simulink model "JuntaFexible"  (R2015a)
settings: Solver=ode4  StartTime=0.0  StopTime=10.0  FixedStep=.001  RelTol=1e-3
settings Model: Creator=Alberto  LastModifiedBy=Jesus
settings DataIOCC: SignalLoggingSaveFormat=ModelDataLogs
settings DebuggingCC: UnderspecifiedInitializationDetection=Classic  MergeDetectMultiDrivingBlocksExec=none  SolverPrmCheckMsg=warning  MultiTaskDSMMsg=warning  MultiTaskCondExecSysMsg=none  StateNameClashWarn=warning

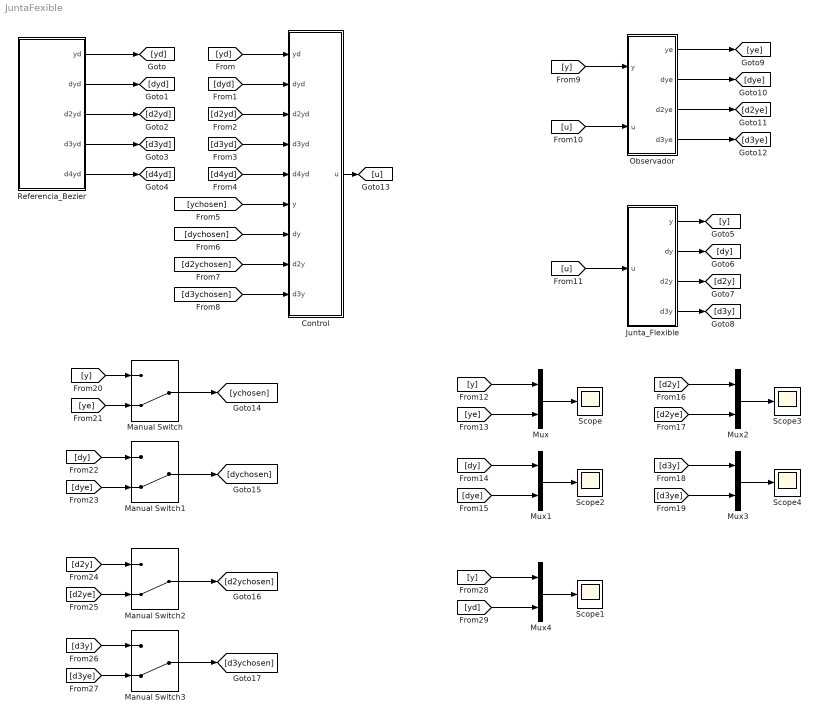
== system JuntaFexible ==
  Control : Subsystem  mask{K=.8, Jl=.1, Jm=.1, Bl=.001, Bm=0.015, z1=5, z2=7.5, w1=150, w2=175}
      mask init:
      | a4=Jl*Jm;
      | a3=Jl*Bm+Jm*Bl;
      | a2=K*(Jl+Jm)+Bl*Bm;
      | a1=K*(Bl+Bm);
      | PD=conv([1 2*z1*w1 w1^2],[1 2*z2*w2 w2^2]);
      | k3=PD(2)-(a3/a4);
      | k2=PD(3)-(a2/a4);
      | k1=PD(4)-(a1/a4);
      | k0=PD(5);
  Junta_Flexible : Subsystem  mask{K=0.8, Jl=.1, Jm=.1, Bl=.001, Bm=.015, y0=.4, dy0=.5, d2y0=0, d3y0=0}
  Manual Switch{,1..3} (4 alike) : ManualSwitch  CurrentSetting=0
  Mux{,1..4} (5 alike) : Mux  Inputs=2
  Observador : Subsystem  mask{K=0.8, Jl=.1, Jm=.1, Bl=.001, Bm=.015, z1o=1, z2o=2, w1o=10, w2o=15}
      mask prompts: z2o "z20"
      mask init:
      | alpha2=K*(Bl+Bm)/(Jl*Jm);
      | alpha3=(K/Jl)+(K/Jm)+((Bl*Bm)/(Jl*Jm));
      | alpha4=(Bl/Jl)+(Bm/Jm);
      | beta=K/(Jl*Jm);
      | PD=conv([1 2*z1o*w1o w1o^2],[1 2*z2o*w2o w2o^2]);
      | lambda3=PD(2)-alpha4;
      | lambda2=PD(3)-alpha3-alpha4*lambda3;
      | lambda1=PD(4)-alpha2-alpha3*lambda3-alpha4*lambda2;
      | lambda0=PD(5)-alpha2*lambda3-alpha3*lambda2-alpha4*lambda1;
  Referencia_Bezier : Subsystem  mask{t1=2, t2=4, y0=.1, yf=10}
      mask prompts: y0 "Valor Inicial"; yf "Valor final"
      mask init:
      | A=[1 -1 1 -1 1;...
      |     5 -6 7 -8 9;...
      |     20 -30 42 -56 72;...
      |     60 -120 210 -336 504;...
      |     120 -360 840 -1680 3024];
      | B=[1;0;0;0;0];
      | x=inv(A)*B;
      | gamma1=x(1)
      | gamma2=x(2)
      | gamma3=x(3)
      | gamma4=x(4)
      | gamma5=x(5)
  Scope{,1..4} (5 alike) : Scope
      Scope settings: YMin=-1  YMax=12
      Scope1 settings: YMin=-1.38898  YMax=11.26544
      Scope2 settings: YMin=-1  YMax=12  SaveName=ScopeData2
      Scope3 settings: YMin=-130.40405  YMax=113.50003  SaveName=ScopeData3
      Scope4 settings: YMin=-367942.44454  YMax=367940.37596  SaveName=ScopeData4
  wires:
  Mux/1 -> Scope/1
  Referencia_Bezier/1(yd) -> [yd]
  Referencia_Bezier/2(dyd) -> [dyd]
  Referencia_Bezier/3(d2yd) -> [d2yd]
  Referencia_Bezier/4(d3yd) -> [d3yd]
  Referencia_Bezier/5(d4yd) -> [d4yd]
  [yd] -> Control/1(yd)
  [dyd] -> Control/2(dyd)
  [d2yd] -> Control/3(d2yd)
  [d3yd] -> Control/4(d3yd)
  [d4yd] -> Control/5(d4yd)
  Junta_Flexible/1(y) -> [y]
  Junta_Flexible/2(dy) -> [dy]
  Junta_Flexible/3(d2y) -> [d2y]
  Junta_Flexible/4(d3y) -> [d3y]
  [ychosen] -> Control/6(y)
  [dychosen] -> Control/7(dy)
  [d2ychosen] -> Control/8(d2y)
  [d3ychosen] -> Control/9(d3y)
  [y] -> Observador/1(y)
  [u] -> Observador/2(u)
  Observador/1(ye) -> [ye]
  Observador/2(dye) -> [dye]
  Observador/3(d2ye) -> [d2ye]
  Observador/4(d3ye) -> [d3ye]
  Control/1(u) -> [u]
  [u] -> Junta_Flexible/1(u)
  [y] -> Mux/1
  [ye] -> Mux/2
  Mux1/1 -> Scope2/1
  [dy] -> Mux1/1
  [dye] -> Mux1/2
  Mux2/1 -> Scope3/1
  [d2y] -> Mux2/1
  [d2ye] -> Mux2/2
  Mux3/1 -> Scope4/1
  [d3y] -> Mux3/1
  [d3ye] -> Mux3/2
  [y] -> Manual Switch/1
  [ye] -> Manual Switch/2
  Manual Switch/1 -> [ychosen]
  Manual Switch1/1 -> [dychosen]
  [dy] -> Manual Switch1/1
  [dye] -> Manual Switch1/2
  Manual Switch2/1 -> [d2ychosen]
  Manual Switch3/1 -> [d3ychosen]
  [d2y] -> Manual Switch2/1
  [d2ye] -> Manual Switch2/2
  [d3y] -> Manual Switch3/1
  [d3ye] -> Manual Switch3/2
  Mux4/1 -> Scope1/1
  [y] -> Mux4/1
  [yd] -> Mux4/2

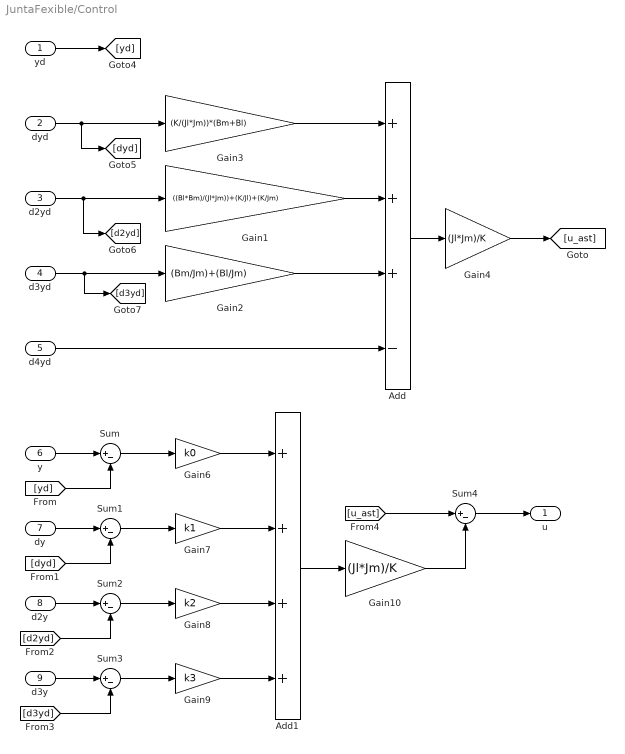
== system JuntaFexible/Control ==
  yd : Inport
  dyd : Inport  Port=2
  d2yd : Inport  Port=3
  d3yd : Inport  Port=4
  d4yd : Inport  Port=5
  y : Inport  Port=6
  dy : Inport  Port=7
  d2y : Inport  Port=8
  d3y : Inport  Port=9
  Add : Sum  Inputs=+++-
  Add1 : Sum  Inputs=++++
  Gain1 : Gain  Gain=((Bl*Bm)/(Jl*Jm))+(K/Jl)+(K/Jm)
  Gain10 : Gain  Gain=(Jl*Jm)/K
  Gain2 : Gain  Gain=(Bm/Jm)+(Bl/Jm)
  Gain3 : Gain  Gain=(K/(Jl*Jm))*(Bm+Bl)
  Gain4 : Gain  Gain=(Jl*Jm)/K
  Gain6 : Gain  Gain=k0
  Gain7 : Gain  Gain=k1
  Gain8 : Gain  Gain=k2
  Gain9 : Gain  Gain=k3
  Sum{,1..4} (5 alike) : Sum  Inputs=|+-
  u : Outport
  wires:
  d3yd/1 -> [d3yd], Gain2/1
  d2yd/1 -> [d2yd], Gain1/1
  Gain1/1 -> Add/2
  Gain2/1 -> Add/3
  Add/1 -> Gain4/1
  dyd/1 -> Gain3/1, [dyd]
  Gain3/1 -> Add/1
  Gain4/1 -> [u_ast]
  yd/1 -> [yd]
  y/1 -> Sum/1
  [yd] -> Sum/2
  Sum/1 -> Gain6/1
  dy/1 -> Sum1/1
  [dyd] -> Sum1/2
  Sum1/1 -> Gain7/1
  d2y/1 -> Sum2/1
  [d2yd] -> Sum2/2
  d3y/1 -> Sum3/1
  [d3yd] -> Sum3/2
  Sum2/1 -> Gain8/1
  Sum3/1 -> Gain9/1
  Gain6/1 -> Add1/1
  Gain7/1 -> Add1/2
  Gain8/1 -> Add1/3
  Gain9/1 -> Add1/4
  Add1/1 -> Gain10/1
  [u_ast] -> Sum4/1
  Gain10/1 -> Sum4/2
  Sum4/1 -> u/1
  d4yd/1 -> Add/4

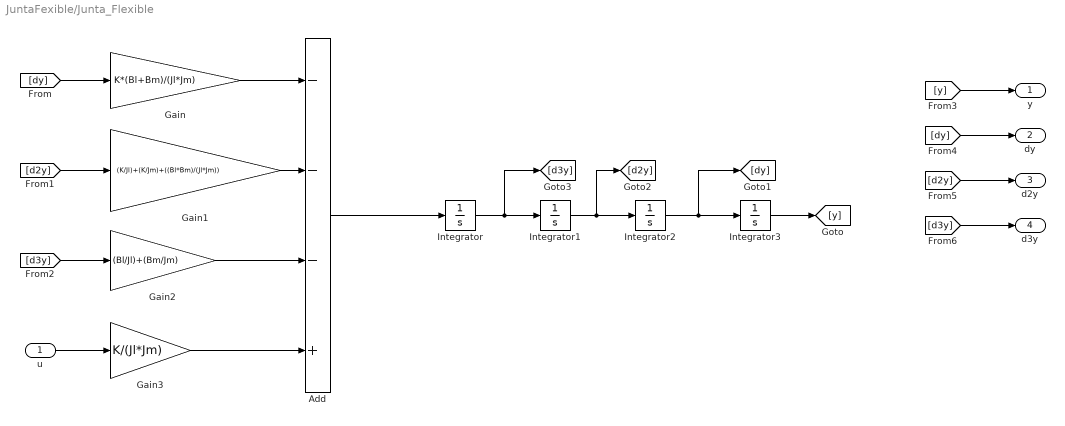
== system JuntaFexible/Junta_Flexible ==
  u : Inport
  Add : Sum  Inputs=---+
  Gain : Gain  Gain=K*(Bl+Bm)/(Jl*Jm)
  Gain1 : Gain  Gain=(K/Jl)+(K/Jm)+((Bl*Bm)/(Jl*Jm))
  Gain2 : Gain  Gain=(Bl/Jl)+(Bm/Jm)
  Gain3 : Gain  Gain=K/(Jl*Jm)
  Integrator : Integrator  InitialCondition=d3y0
  Integrator1 : Integrator  InitialCondition=d2y0
  Integrator2 : Integrator  InitialCondition=dy0
  Integrator3 : Integrator  InitialCondition=y0
  y : Outport
  dy : Outport  Port=2
  d2y : Outport  Port=3
  d3y : Outport  Port=4
  wires:
  Integrator3/1 -> [y]
  Integrator/1 -> [d3y], Integrator1/1
  [d3y] -> d3y/1
  Gain/1 -> Add/1
  [y] -> y/1
  Integrator2/1 -> [dy], Integrator3/1
  Integrator1/1 -> [d2y], Integrator2/1
  [dy] -> Gain/1
  Gain2/1 -> Add/3
  Gain3/1 -> Add/4
  Gain1/1 -> Add/2
  [dy] -> dy/1
  [d2y] -> d2y/1
  [d2y] -> Gain1/1
  Add/1 -> Integrator/1
  [d3y] -> Gain2/1
  u/1 -> Gain3/1

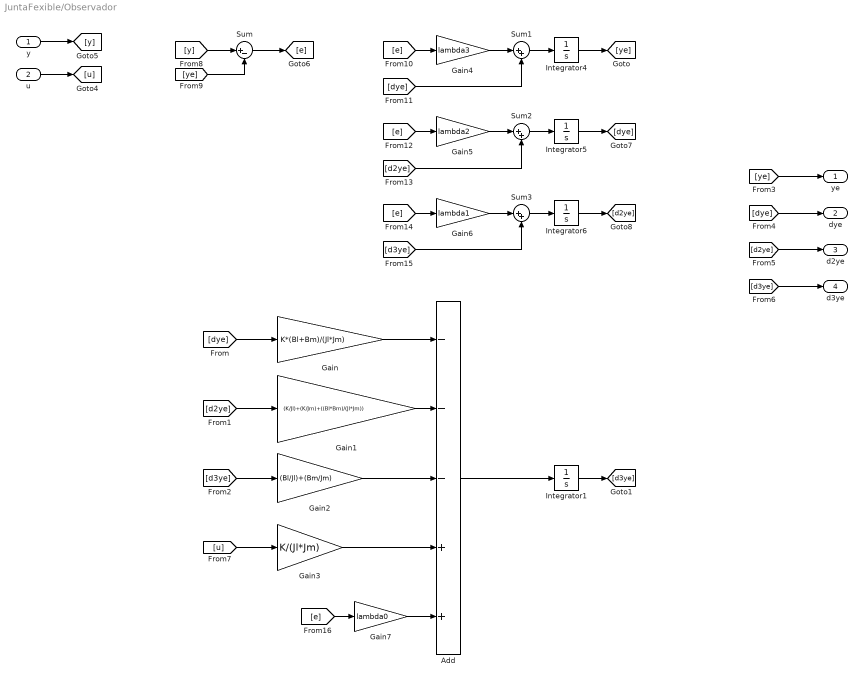
== system JuntaFexible/Observador ==
  y : Inport
  u : Inport  Port=2
  Add : Sum  Inputs=---++
  Gain : Gain  Gain=K*(Bl+Bm)/(Jl*Jm)
  Gain1 : Gain  Gain=(K/Jl)+(K/Jm)+((Bl*Bm)/(Jl*Jm))
  Gain2 : Gain  Gain=(Bl/Jl)+(Bm/Jm)
  Gain3 : Gain  Gain=K/(Jl*Jm)
  Gain4 : Gain  Gain=lambda3
  Gain5 : Gain  Gain=lambda2
  Gain6 : Gain  Gain=lambda1
  Gain7 : Gain  Gain=lambda0
  Integrator{1,4..6} (4 alike) : Integrator
  Sum : Sum  Inputs=|+-
  Sum1 : Sum  Inputs=|++
  Sum2 : Sum  Inputs=|++
  Sum3 : Sum  Inputs=|++
  ye : Outport
  dye : Outport  Port=2
  d2ye : Outport  Port=3
  d3ye : Outport  Port=4
  wires:
  [d3ye] -> Gain2/1
  [d2ye] -> Gain1/1
  [d2ye] -> d2ye/1
  [dye] -> dye/1
  Gain1/1 -> Add/2
  Gain3/1 -> Add/4
  Gain2/1 -> Add/3
  [dye] -> Gain/1
  [ye] -> ye/1
  Gain/1 -> Add/1
  [d3ye] -> d3ye/1
  [u] -> Gain3/1
  u/1 -> [u]
  y/1 -> [y]
  Integrator4/1 -> [ye]
  [y] -> Sum/1
  [ye] -> Sum/2
  Sum/1 -> [e]
  [e] -> Gain4/1
  [dye] -> Sum1/2
  Sum1/1 -> Integrator4/1
  Gain4/1 -> Sum1/1
  Integrator5/1 -> [dye]
  [e] -> Gain5/1
  [d2ye] -> Sum2/2
  Sum2/1 -> Integrator5/1
  Gain5/1 -> Sum2/1
  Integrator6/1 -> [d2ye]
  [e] -> Gain6/1
  [d3ye] -> Sum3/2
  Sum3/1 -> Integrator6/1
  Gain6/1 -> Sum3/1
  Add/1 -> Integrator1/1
  [e] -> Gain7/1
  Gain7/1 -> Add/5
  Integrator1/1 -> [d3ye]

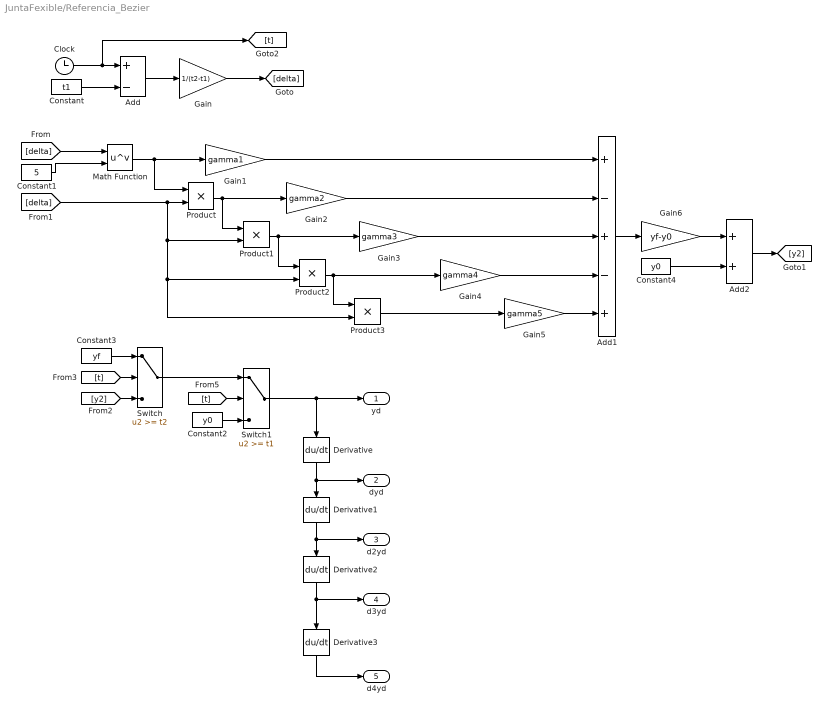
== system JuntaFexible/Referencia_Bezier ==
  Add : Sum  Inputs=+-
  Add1 : Sum  Inputs=+-+-+
  Add2 : Sum
  Clock : Clock
  Constant : Constant  Value=t1
  Constant1 : Constant  Value=5
  Constant2 : Constant  Value=y0
  Constant3 : Constant  Value=yf
  Constant4 : Constant  Value=y0
  Derivative{,1..3} (4 alike) : Derivative
  Gain : Gain  Gain=1/(t2-t1)
  Gain1 : Gain  Gain=gamma1
  Gain2 : Gain  Gain=gamma2
  Gain3 : Gain  Gain=gamma3
  Gain4 : Gain  Gain=gamma4
  Gain5 : Gain  Gain=gamma5
  Gain6 : Gain  Gain=yf-y0
  Math Function : Math  Operator=pow  SaturateOnIntegerOverflow=on
  Product{,1..3} (4 alike) : Product  RndMeth=Zero
  Switch : Switch  Threshold=t2
  Switch1 : Switch  Threshold=t1
  yd : Outport
  dyd : Outport  Port=2
  d2yd : Outport  Port=3
  d3yd : Outport  Port=4
  d4yd : Outport  Port=5
  wires:
  Constant/1 -> Add/2
  Clock/1 -> Add/1, [t]
  Add/1 -> Gain/1
  Gain/1 -> [delta]
  [delta] -> Math Function/1
  Constant1/1 -> Math Function/2
  Math Function/1 -> Product/1, Gain1/1
  [delta] -> Product/2, Product1/2, Product2/2, Product3/2
  Product/1 -> Product1/1, Gain2/1
  Product1/1 -> Product2/1, Gain3/1
  Product2/1 -> Product3/1, Gain4/1
  Product3/1 -> Gain5/1
  Gain5/1 -> Add1/5
  Gain1/1 -> Add1/1
  Gain2/1 -> Add1/2
  Gain3/1 -> Add1/3
  Gain4/1 -> Add1/4
  Add1/1 -> Gain6/1
  Constant3/1 -> Switch/1
  [y2] -> Switch/3
  [t] -> Switch/2
  Switch/1 -> Switch1/1
  Constant2/1 -> Switch1/3
  [t] -> Switch1/2
  Switch1/1 -> Derivative/1, yd/1
  Gain6/1 -> Add2/1
  Constant4/1 -> Add2/2
  Add2/1 -> [y2]
  Derivative/1 -> dyd/1, Derivative1/1
  Derivative1/1 -> d2yd/1, Derivative2/1
  Derivative2/1 -> Derivative3/1, d3yd/1
  Derivative3/1 -> d4yd/1
